simulink model "mngmdl"  (Simulink 7.6)
settings: Solver=FixedStepDiscrete  SolverMode=SingleTasking  StartTime=TIME(1)  StopTime=TIME(end)  FixedStep=SIMSTEP  RelTol=1e-3
model workspace (MAT data in the model file):
  autoc_mdd_data01.esubassyinfo_cfg.cd_brdgname = 'cpsmdlbrg'
  autoc_mdd_data01.esubassyinfo_cfg.cd_exinc = 'on'
  autoc_mdd_data01.esubassyinfo_cfg.cd_chknan = 'on'
  autoc_mdd_data01.esubassyinfo_cfg.cd_geninit = 'on'
  autoc_mdd_data01.esubassyinfo_cfg.cd_fxpimp = 'on'
  autoc_mdd_data01.esubassyinfo_cfg.cd_fixgd = 'on'
  autoc_mdd_data01.esubassyinfo_cfg.cd_models = '.\cpsaflfb.mdl|.\cpsgain.mdl|.\cpsmbtfb.mdl|.\cpsmfb.mdl|.\cpsparam.mdl'
  autoc_mdd_data01.esubassyinfo_cfg.cd_optm_copy = 'off'
  autoc_mdd_data01.esubassyinfo_cfg.cd_optm_nocopy = 'on'
  autoc_mdd_data01.esubassyinfo_cfg.cd_userdefspec = '[-------- 仕様書用 --------]
    | [fram section id]
    | u4g_GSFRAM_CPS_ID
    | [model function]
    | pwon:cpsparam_pwon();
    | pwon:cpsgain_pwon();
    | pwon:cpsmfb_pwon();
    | pwon:cpsaflfb_pwon();
    | pwon:cpsmbtfb_pwon();
    | crank144:cpsparam_crank144();
    | crank144:cpsgain_crank144();
    | crank144:cpsmfb_crank144();
    | crank144:cpsaflfb_crank144();
    | crank144:cpsmbtfb_crank144();
    | [task input]
    | [task output]
    | [output trigger c]
    | [nan recover]
    | [bridge const]
    | [auto counter]
    | [const]
    | [sram]'
  autoc_mdd_data01.esubassyinfo_cfg.cd_userdef_ecuimp : char (value not decoded)
  autoc_mdd_data01.egencode_cfg.cd_stclass_mat = 'rule'
  autoc_mdd_data01.egencode_cfg.cd_option_mode = 'strict'
  autoc_mdd_data01.egencode_cfg.cd_stclass_dsm = 'colored'
  autoc_mdd_data01.egencode_cfg.cd_autoset_simprm = 'on'
  autoc_mdd_data01.egencode_cfg.cd_autoset_mat = 'on'
  autoc_mdd_data01.egencode_cfg.cd_autoset_dsm = 'on'
  autoc_mdd_data01.egencode_cfg.cd_postprocess = 'on'
  autoc_mdd_data01.egencode_cfg.cd_sw_cmatm = 'off'
  autoc_mdd_data01.egencode_cfg.cd_prepro_mdlchk = 'on'
  autoc_mdd_data01.egencode_cfg.cd_cmat_comment = 'on'
  autoc_mdd_data01.egencode_cfg.cd_towscsv_sw = 'off'
  autoc_mdd_data01.egencode_cfg.cd_towscsv_dlg = ''
  autoc_mdd_data01.egencode_cfg.cd_varicodecsv_dlg = ''
  autoc_mdd_data01.egencode_cfg.cd_gencode_lcmat = 'lcmat'
  autoc_mdd_data01.egencode_cfg.cd_option_mode_for_sim = 'off'
  autoc_mdd_data01.egencode_cfg.cd_numexp_opt = 'off'
  autoc_mdd_data01.egencode_cfg.cd_pragmasection = 'cpsmdl_data'
  autoc_mdd_data01.egencode_cfg.cd_returncode_opt = 'off'
  autoc_mdd_data01.egencode_cfg.cd_module_name = 'cpsmdl'
  autoc_mdd_data01.egencode_cfg.cd_expansion_include = '#include "./esrc_cpsmdlbrg.h"'
  autoc_mdd_data01.egencode_cfg.cd_sim_datatype_mode = 'double'
  autoc_mdd_data01.egencode_cfg.cd_mat_cmplsw = 'JEMAT_AUTOC == u1g_EJCC_USE'
  autoc_mdd_data01.egencode_cfg.cd_mon_cmplsw = 'JEMAT_AUTOC == u1g_EJCC_USE'
  autoc_mdd_data01.evaluetows_cfg.cd_ejccpath = ''
  autoc_mdd_data01.evaluetows_cfg.cd_valuews_path = ''
  autoc_mdd_data01.a_cst = []
  autoc_mdd_data01.SIMSTEP = []
  autoc_mdd_data01.MAX_CYL = []
  autoc_mdd_data01.cpsdata_low1 = []
  autoc_mdd_data01.cpsdata_low0 = []
  autoc_mdd_data01.cpsdata_hih1 = []
  autoc_mdd_data01.cpsdata_abs_hih0 = []
  autoc_mdd_data01.cpsdata_hih2 = []
  autoc_mdd_data01.cpsdata_abs_hih1 = []
  autoc_mdd_data01.cpsdata_abs_hih2 = []
  autoc_mdd_data01.cpsdata_hih0 = []
  autoc_mdd_data01.cpsdata_low2 = []
  autoc_mdd_data01.arg_adcn = []
  autoc_mdd_data01.GCIAD_ADCNO0 = []
  autoc_mdd_data01.GACPSCRNK_5CA4CYCLE = []
  autoc_mdd_data01.ON = []
  autoc_mdd_data01.geadd_gepim = []
  autoc_mdd_data01.geadd_gevg = []
  autoc_mdd_data01.geadd_gecps1h = []
  autoc_mdd_data01.geadd_gecps2h = []
  autoc_mdd_data01.geadd_gecps3h = []
  autoc_mdd_data01.geadd_gecps4h = []
  autoc_mdd_data01.geadd_gecps1l = []
  autoc_mdd_data01.geadd_gecps2l = []
  autoc_mdd_data01.geadd_gecps3l = []
  autoc_mdd_data01.geadd_gecps4l = []
  autoc_mdd_data01.revtdc = []
  autoc_mdd_data01.gacpscrnk_cps1 = []
  autoc_mdd_data01.gacpscrnk_cps2 = []
  autoc_mdd_data01.gacpscrnk_cps4 = []
  autoc_mdd_data01.gacpscrnk_cps6 = []
  autoc_mdd_data01.gacpscrnk_cps3 = []
  autoc_mdd_data01.gacpscrnk_cps0 = []
  autoc_mdd_data01.gacpscrnk_cps7 = []
  autoc_mdd_data01.gacpscrnk_cps9 = []
  autoc_mdd_data01.gacpscrnk_cps8 = []
  autoc_mdd_data01.gacpscrnk_cps5 = []
  autoc_mdd_data01.gacpscrnk_cps_idx1 = []
  autoc_mdd_data01.gacpscrnk_cps_idx2 = []
  autoc_mdd_data01.gacpscrnk_cps_result = []
  autoc_mdd_data01.Parameter145 = []
  autoc_mdd_data01.DSM405 = []
  autoc_mdd_data01.DSM406 = []
  autoc_mdd_data01.DSM407 = []
  autoc_mdd_data01.DSM408 = []
  autoc_mdd_data01.DSM409 = []
  autoc_mdd_data01.DSM410 = []
  autoc_mdd_data01.DSM411 = []
  autoc_mdd_data01.DSM412 = []
  autoc_mdd_data01.DSM413 = []
  autoc_mdd_data01.DSM414 = []
  autoc_mdd_data01.DSM39 = []
  autoc_mdd_data01.DSM51 = []
  autoc_mdd_data01.DSM53 = []
  autoc_mdd_data01.DSM62 = []
  autoc_mdd_data01.DSM72 = []
  autoc_mdd_data01.DSM77 = []
  autoc_mdd_data01.DSM79 = []
  autoc_mdd_data01.DSM80 = []
  autoc_mdd_data01.DSM81 = []
values from neighbouring files (symbols this model uses):
  SIMSTEP = 0.0001024    [scr_simdata_all.mat]
Description:
  | AutoCodeGenerator:Version 1.01.A;
settings Model: autoc_cdm_savetype=ModelWorkspace  autoc_cdm_name=autoc_mdd_data01  autoc_current_model=mngmdl  autoc_dsminitmode=spec  Creator=905900  LastModifiedBy=fukudak
settings OptimizationCC: InlineParams=on  InlineInvariantSignals=on  UseTempVars=on  InitFltsAndDblsToZero=on  OptimizeModelRefInitCode=on  LifeSpan=1
settings DebuggingCC: ConsistencyChecking=warning  ArrayBoundsChecking=warning  SignalInfNanChecking=warning  AlgebraicLoopMsg=error  SaveWithParameterizedLinksMsg=none  CheckExecutionContextPreStartOutputMsg=on  CheckExecutionContextRuntimeOutputMsg=on  TimeAdjustmentMsg=warning  SolverPrmCheckMsg=none  InheritedTsInSrcMsg=none  MultiTaskDSMMsg=warning  SingleTaskRateTransMsg=warning  TasksWithSamePriorityMsg=none  IntegerOverflowMsg=error  VectorMatrixConversionMsg=warning  UnconnectedInputMsg=error  UnconnectedOutputMsg=error  UnconnectedLineMsg=error  UniqueDataStoreMsg=error  BusObjectLabelMismatch=error  RootOutportRequireBusObject=error  ModelReferenceIOMsg=warning  ModelReferenceIOMismatchMessage=warning  StrictBusMsg=Warning
settings HardwareCC: ProdIntDivRoundTo=Floor  ProdEndianess=LittleEndian  ProdHWDeviceType=Specified  TargetHWDeviceType=32-bit Generic  ProdEqTarget=off
settings ModelReferenceCC: ModelReferenceNumInstancesAllowed=Single
settings RTWCC: SystemTargetFile=ert.tlc  GenCodeOnly=on  TemplateMakefile=ert_default_tmf  Description=Real-Time Workshop Embedded Coder (no auto configuration)  RTWVerbose=off  ProcessScript=ert_make_rtw_hook
settings CodeAppCC: ForceParamTrailComments=on  IgnoreCustomStorageClasses=off
settings ERTTargetCC: TargetFcnLib=ansi_tfl_tmw.mat  MultiwordLength=2048  GenerateSampleERTMain=on  InlinedParameterPlacement=NonHierarchical  ERTCustomFileTemplate=example_file_process.tlc  ConvertIfToSwitch=off

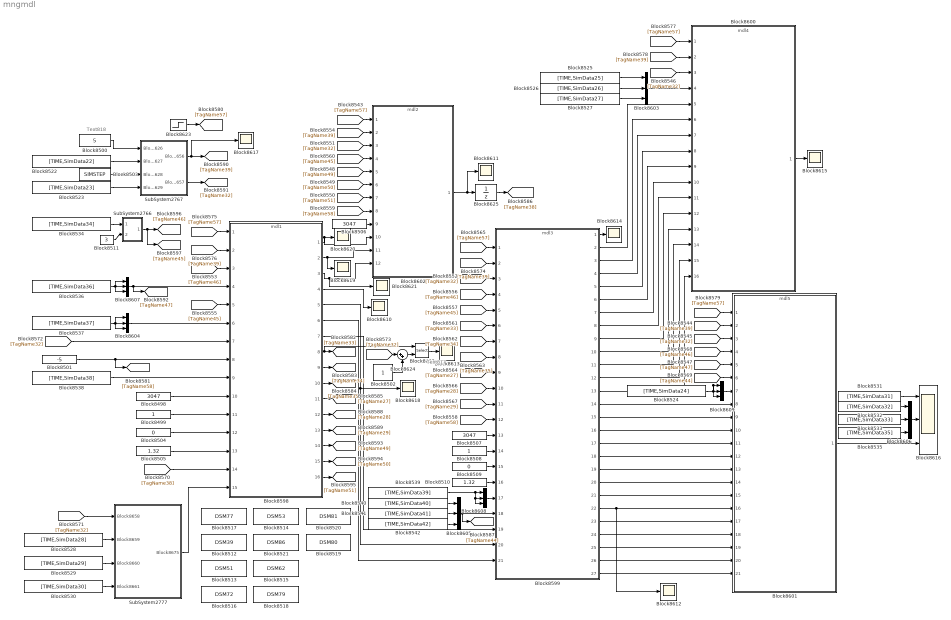
== system mngmdl ==
  note: Text818
  note: Text817
  Block8498 : Constant  Value=3047  OutDataTypeStr=double  SampleTime=SIMSTEP
  Block8499 : Constant  OutDataTypeStr=double  SampleTime=SIMSTEP
  Block8500 : Constant  Value=5  OutDataTypeStr=double  SampleTime=-1
  Block8501 : Constant  Value=-5  OutDataTypeStr=double  SampleTime=SIMSTEP
  Block8502 : Constant  OutDataTypeStr=double  SampleTime=-1
  Block8503 : Constant  Value=SIMSTEP  OutDataTypeStr=double  SampleTime=-1
  Block8504 : Constant  Value=0  OutDataTypeStr=double  SampleTime=SIMSTEP
  Block8505 : Constant  Value=1.32  OutDataTypeStr=double  SampleTime=SIMSTEP
  Block8506 : Constant  Value=3047  OutDataTypeStr=double  SampleTime=-1
  Block8507 : Constant  Value=3047  OutDataTypeStr=double  SampleTime=SIMSTEP
  Block8508 : Constant  OutDataTypeStr=double  SampleTime=SIMSTEP
  Block8509 : Constant  Value=0  OutDataTypeStr=double  SampleTime=SIMSTEP
  Block8510 : Constant  Value=1.32  OutDataTypeStr=double  SampleTime=SIMSTEP
  Block8511 : Constant  Value=3  OutDataTypeStr=double  SampleTime=-1
  Block8512 : DataStoreMemory  DataStoreName=DSM39  InitialValue=[0 0 0 0 0 0 0 0 0 0 0 0 0 0 0 0 0 0 0 0 0 0 0 0 0 0 0 0 0 0 0 0 0 0 0 0 0 0 0 0 0 0 0 0 0 0 0 0 0 0 0 0 0 0 0 0 0 0 0 0 0 0 0 0 0 0 0 0 0 0 0 0 0 0 0 0 0 0 0 0 0 0 0 0 0 0 0 0 0 0 0 0 0 0 0 0 0 0 0 0 0 0 0 0 0 0 0 0 0 0 0 0 0 0 0 0 0 0 0 0 0 0 0 0 0 0 0 0 0 0 0 0 0 0 0 0 0 0 0 0 0 0 0 0]  OutDataTypeStr=double
  Block8513 : DataStoreMemory  DataStoreName=DSM51  InitialValue=[0 0 0 0 0 0 0 0 0 0 0 0 0 0 0 0 0 0 0 0 0 0 0 0 0 0 0 0 0 0 0 0 0 0 0 0 0 0 0 0 0 0 0 0 0 0 0 0 0 0 0 0 0 0 0 0 0 0 0 0 0 0 0 0 0 0 0 0 0 0 0 0 0 0 0 0 0 0 0 0 0 0 0 0 0 0 0 0 0 0 0 0 0 0 0 0 0 0 0 0 0 0 0 0 0 0 0 0 0 0 0 0 0 0 0 0 0 0 0 0 0 0 0 0 0 0 0 0 0 0 0 0 0 0 0 0 0 0 0 0 0 0 0 0]  OutDataTypeStr=double
  Block8514 : DataStoreMemory  DataStoreName=DSM53  InitialValue=[0 0 0 0 0 0 0 0 0 0 0 0 0 0 0 0 0 0 0 0 0 0 0 0 0 0 0 0 0 0 0 0 0 0 0 0 0 0 0 0 0 0 0 0 0 0 0 0 0 0 0 0 0 0 0 0 0 0 0 0 0 0 0 0 0 0 0 0 0 0 0 0 0 0 0 0 0 0 0 0 0 0 0 0 0 0 0 0 0 0 0 0 0 0 0 0 0 0 0 0 0 0 0 0 0 0 0 0 0 0 0 0 0 0 0 0 0 0 0 0 0 0 0 0 0 0 0 0 0 0 0 0 0 0 0 0 0 0 0 0 0 0 0 0]  OutDataTypeStr=double
  Block8515 : DataStoreMemory  DataStoreName=DSM62  InitialValue=[0 0 0 0 0 0 0 0 0 0 0 0 0 0 0 0 0 0 0 0 0 0 0 0 0 0 0 0 0 0 0 0 0 0 0 0 0 0 0 0 0 0 0 0 0 0 0 0 0 0 0 0 0 0 0 0 0 0 0 0 0 0 0 0 0 0 0 0 0 0 0 0 0 0 0 0 0 0 0 0 0 0 0 0 0 0 0 0 0 0 0 0 0 0 0 0 0 0 0 0 0 0 0 0 0 0 0 0 0 0 0 0 0 0 0 0 0 0 0 0 0 0 0 0 0 0 0 0 0 0 0 0 0 0 0 0 0 0 0 0 0 0 0 0]  OutDataTypeStr=double
  Block8516 : DataStoreMemory  DataStoreName=DSM72  InitialValue=[0 0 0 0 0 0 0 0 0 0 0 0 0 0 0 0 0 0 0 0 0 0 0 0 0 0 0 0 0 0 0 0 0 0 0 0 0 0 0 0 0 0 0 0 0 0 0 0 0 0 0 0 0 0 0 0 0 0 0 0 0 0 0 0 0 0 0 0 0 0 0 0 0 0 0 0 0 0 0 0 0 0 0 0 0 0 0 0 0 0 0 0 0 0 0 0 0 0 0 0 0 0 0 0 0 0 0 0 0 0 0 0 0 0 0 0 0 0 0 0 0 0 0 0 0 0 0 0 0 0 0 0 0 0 0 0 0 0 0 0 0 0 0 0]  OutDataTypeStr=double
  Block8517 : DataStoreMemory  DataStoreName=DSM77  InitialValue=[0 0 0 0 0 0 0 0 0 0 0 0 0 0 0 0 0 0 0 0 0 0 0 0 0 0 0 0 0 0 0 0 0 0 0 0 0 0 0 0 0 0 0 0 0 0 0 0 0 0 0 0 0 0 0 0 0 0 0 0 0 0 0 0 0 0 0 0 0 0 0 0 0 0 0 0 0 0 0 0 0 0 0 0 0 0 0 0 0 0 0 0 0 0 0 0 0 0 0 0 0 0 0 0 0 0 0 0 0 0 0 0 0 0 0 0 0 0 0 0 0 0 0 0 0 0 0 0 0 0 0 0 0 0 0 0 0 0 0 0 0 0 0 0]  OutDataTypeStr=double
  Block8518 : DataStoreMemory  DataStoreName=DSM79  InitialValue=[0 0 0 0 0 0 0 0 0 0 0 0 0 0 0 0 0 0 0 0 0 0 0 0 0 0 0 0 0 0 0 0 0 0 0 0 0 0 0 0 0 0 0 0 0 0 0 0 0 0 0 0 0 0 0 0 0 0 0 0 0 0 0 0 0 0 0 0 0 0 0 0 0 0 0 0 0 0 0 0 0 0 0 0 0 0 0 0 0 0 0 0 0 0 0 0 0 0 0 0 0 0 0 0 0 0 0 0 0 0 0 0 0 0 0 0 0 0 0 0 0 0 0 0 0 0 0 0 0 0 0 0 0 0 0 0 0 0 0 0 0 0 0 0]  OutDataTypeStr=double
  Block8519 : DataStoreMemory  DataStoreName=DSM80  InitialValue=[0 0 0 0 0 0 0 0 0 0 0 0 0 0 0 0 0 0 0 0 0 0 0 0 0 0 0 0 0 0 0 0 0 0 0 0 0 0 0 0 0 0 0 0 0 0 0 0 0 0 0 0 0 0 0 0 0 0 0 0 0 0 0 0 0 0 0 0 0 0 0 0 0 0 0 0 0 0 0 0 0 0 0 0 0 0 0 0 0 0 0 0 0 0 0 0 0 0 0 0 0 0 0 0 0 0 0 0 0 0 0 0 0 0 0 0 0 0 0 0 0 0 0 0 0 0 0 0 0 0 0 0 0 0 0 0 0 0 0 0 0 0 0 0]  OutDataTypeStr=double
  Block8520 : DataStoreMemory  DataStoreName=DSM81  InitialValue=[0 0 0 0 0 0 0 0 0 0 0 0 0 0 0 0 0 0 0 0 0 0 0 0 0 0 0 0 0 0 0 0 0 0 0 0 0 0 0 0 0 0 0 0 0 0 0 0 0 0 0 0 0 0 0 0 0 0 0 0 0 0 0 0 0 0 0 0 0 0 0 0 0 0 0 0 0 0 0 0 0 0 0 0 0 0 0 0 0 0 0 0 0 0 0 0 0 0 0 0 0 0 0 0 0 0 0 0 0 0 0 0 0 0 0 0 0 0 0 0 0 0 0 0 0 0 0 0 0 0 0 0 0 0 0 0 0 0 0 0 0 0 0 0]  OutDataTypeStr=double
  Block8521 : DataStoreMemory  DataStoreName=DSM86  InitialValue=[0 0 0 0 0 0 0 0 0 0 0 0 0 0 0 0 0 0 0 0 0 0 0 0 0 0 0 0 0 0 0 0 0 0 0 0 0 0 0 0 0 0 0 0 0 0 0 0 0 0 0 0 0 0 0 0 0 0 0 0 0 0 0 0 0 0 0 0 0 0 0 0 0 0 0 0 0 0 0 0 0 0 0 0 0 0 0 0 0 0 0 0 0 0 0 0 0 0 0 0 0 0 0 0 0 0 0 0 0 0 0 0 0 0 0 0 0 0 0 0 0 0 0 0 0 0 0 0 0 0 0 0 0 0 0 0 0 0 0 0 0 0 0 0]  OutDataTypeStr=double
  Block8522 : FromWorkspace  VariableName=[TIME,SimData22]  SampleTime=SIMSTEP
  Block8523 : FromWorkspace  VariableName=[TIME,SimData23]  SampleTime=SIMSTEP  Interpolate=off  OutputAfterFinalValue=Holding final value
  Block8524 : FromWorkspace  VariableName=[TIME,SimData24]  SampleTime=SIMSTEP
  Block8525 : FromWorkspace  VariableName=[TIME,SimData25]  SampleTime=SIMSTEP
  Block8526 : FromWorkspace  VariableName=[TIME,SimData26]  SampleTime=SIMSTEP
  Block8527 : FromWorkspace  VariableName=[TIME,SimData27]  SampleTime=SIMSTEP
  Block8528 : FromWorkspace  VariableName=[TIME,SimData28]  SampleTime=SIMSTEP
  Block8529 : FromWorkspace  VariableName=[TIME,SimData29]  SampleTime=SIMSTEP
  Block8530 : FromWorkspace  VariableName=[TIME,SimData30]  SampleTime=SIMSTEP
  Block8531 : FromWorkspace  VariableName=[TIME,SimData31]  SampleTime=SIMSTEP
  Block8532 : FromWorkspace  VariableName=[TIME,SimData32]  SampleTime=SIMSTEP
  Block8533 : FromWorkspace  VariableName=[TIME,SimData33]  SampleTime=SIMSTEP
  Block8534 : FromWorkspace  VariableName=[TIME,SimData34]  SampleTime=SIMSTEP
  Block8535 : FromWorkspace  VariableName=[TIME,SimData35]  SampleTime=SIMSTEP
  Block8536 : FromWorkspace  VariableName=[TIME,SimData36]  SampleTime=SIMSTEP
  Block8537 : FromWorkspace  VariableName=[TIME,SimData37]  SampleTime=SIMSTEP
  Block8538 : FromWorkspace  VariableName=[TIME,SimData38]  SampleTime=SIMSTEP
  Block8539 : FromWorkspace  VariableName=[TIME,SimData39]  SampleTime=SIMSTEP
  Block8540 : FromWorkspace  VariableName=[TIME,SimData40]  SampleTime=SIMSTEP
  Block8541 : FromWorkspace  VariableName=[TIME,SimData41]  SampleTime=SIMSTEP
  Block8542 : FromWorkspace  VariableName=[TIME,SimData42]  SampleTime=SIMSTEP
  Block8598 : ModelReference  Priority=2  ModelNameDialog=mdl1  SimulationMode=Normal  ModelReferenceVersion=1.40  CopyOfModelName=mdl1
      settings: AttributesFormatString=Attribute2295
  Block8599 : ModelReference  Priority=4  ModelNameDialog=mdl3  SimulationMode=Normal  ModelReferenceVersion=1.21  CopyOfModelName=mdl3
      settings: AttributesFormatString=Attribute2296
  Block8600 : ModelReference  Priority=5  ModelNameDialog=mdl4  SimulationMode=Normal  ModelReferenceVersion=1.15  CopyOfModelName=mdl4
      settings: AttributesFormatString=Attribute2297
  Block8601 : ModelReference  Priority=6  ModelNameDialog=mdl5  SimulationMode=Normal  ModelReferenceVersion=1.17  CopyOfModelName=mdl5
      settings: AttributesFormatString=Attribute2298
  Block8602 : ModelReference  Priority=3  ModelNameDialog=mdl2  SimulationMode=Normal  ModelReferenceVersion=1.14  CopyOfModelName=mdl2
      settings: AttributesFormatString=Attribute2299
  Block{8603..8609} (7 alike) : Mux  Inputs=3
  Block{8610..8615,8617..8621} (11 alike) : Scope
      Block8611 settings: YMin=0.95  YMax=1.05
      Block8612 settings: YMin=-0.00475  YMax=-0.0015  SaveName=ScopeData2
      Block8613 settings: YMin=0.125  YMax=0.65  SaveName=ScopeData9
      Block8614 settings: YMin=-1  YMax=1  SaveName=ScopeData10
      Block8615 settings: SaveName=ScopeData11
      Block8617 settings: YMin=0  YMax=1  SaveName=ScopeData4
      Block8618 settings: SaveName=ScopeData5
      Block8619 settings: TimeRange=42.74809160305345  YMin=-0.4345238095238095  YMax=0.2202380952380953  SaveName=ScopeData6
      Block8620 settings: SaveName=ScopeData7
      Block8621 settings: SaveName=ScopeData8
  Block8616 : Scope  NumInputPorts=3
      settings: TimeRange=70  YMin=400~0.8~4.5  YMax=2200~1.8~5.5  SaveName=ScopeData3
  Block8622 : Selector  IndexOptions=Index vector (port)  Indices=[1 3]  OutputSizes=1
  Block8623 : Step  Time=SIMSTEP  SampleTime=SIMSTEP
  Block8624 : Sum  Inputs=|++  OutDataTypeStr=double  RndMeth=Zero  SaturateOnIntegerOverflow=on  InputSameDT=on
  Block8625 : UnitDelay  SampleTime=-1
  SubSystem2766 : Subsystem
  SubSystem2767 : Subsystem
  SubSystem2777 : Subsystem  RTWFileName=eset_real
      settings: AttributesFormatString=Attribute2311  RTWFcnNameOpts=Use subsystem name
  wires:
  Block8598/4 -> Block8610/1
  Block8599/1 -> Block8614/1
  Block8600/1 -> Block8615/1
  Block8599/2 -> Block8600/5
  Block8599/3 -> Block8600/6
  Block8599/4 -> Block8600/7
  Block8599/5 -> Block8600/8
  Block8599/6 -> Block8600/9
  Block8599/7 -> Block8600/10
  Block8599/8 -> Block8600/11
  Block8599/9 -> Block8600/12
  Block8599/10 -> Block8600/13
  Block8599/11 -> Block8600/14
  Block8599/12 -> Block8600/15
  Block8599/13 -> Block8600/16
  Block8599/14 -> Block8601/8
  Block8599/15 -> Block8601/9
  Block8599/16 -> Block8601/10
  Block8599/17 -> Block8601/11
  Block8599/18 -> Block8601/12
  Block8599/19 -> Block8601/13
  Block8599/20 -> Block8601/14
  Block8599/21 -> Block8601/15
  Block8599/22 -> Block8601/16, Block8612/1
  Block8599/23 -> Block8601/17
  Block8599/24 -> Block8601/18
  Block8599/25 -> Block8601/19
  Block8599/26 -> Block8601/20
  Block8599/27 -> Block8601/21
  Block8598/1 -> Block8620/1, Block8602/10
  Block8598/2 -> Block8619/1, Block8602/11
  Block8598/3 -> Block8602/12, Block8621/1
  Block8598/7 -> Block8599/19
  Block8598/5 -> Block8599/20, Block8618/1
  Block8598/6 -> Block8599/21
  Block8607/1 -> Block8598/4, [TagName47]
  Block8604/1 -> Block8598/6
  Block8501/1 -> [TagName58], Block8598/8
  Block8506/1 -> Block8602/9
  [TagName58] -> Block8602/8
  Block8623/1 -> [TagName57]
  [TagName57] -> Block8598/1
  [TagName39] -> Block8598/2
  [TagName57] -> Block8602/1
  [TagName39] -> Block8602/2
  [TagName57] -> Block8599/1
  [TagName39] -> Block8599/2
  [TagName57] -> Block8600/1
  [TagName39] -> Block8600/2
  Block8525/1 -> Block8603/1
  Block8526/1 -> Block8603/2
  Block8527/1 -> Block8603/3
  Block8603/1 -> Block8600/4
  [TagName57] -> Block8601/1
  [TagName39] -> Block8601/2
  [TagName32] -> Block8601/3
  [TagName32] -> Block8600/3
  [TagName44] -> Block8601/6
  [TagName47] -> Block8601/5
  [TagName49] -> Block8602/5
  [TagName51] -> Block8602/7
  [TagName50] -> Block8602/6
  [TagName32] -> Block8602/3
  [TagName32] -> Block8599/3
  Block8534/1 -> SubSystem2766/1(Scalar)
  [TagName46] -> Block8598/3
  [TagName45] -> Block8598/5
  [TagName46] -> Block8599/4
  [TagName45] -> Block8599/5
  [TagName58] -> Block8599/12
  Block8507/1 -> Block8599/13
  Block8508/1 -> Block8599/14
  Block8509/1 -> Block8599/15
  Block8510/1 -> Block8599/16
  [TagName45] -> Block8602/4
  Block8540/1 -> Block8605/1
  Block8541/1 -> Block8605/2
  Block8542/1 -> Block8605/3
  Block8605/1 -> Block8599/18, [TagName44]
  [TagName33] -> Block8599/6
  [TagName35] -> Block8599/8
  [TagName34] -> Block8599/7
  [TagName27] -> Block8599/9
  [TagName28] -> Block8599/10
  [TagName29] -> Block8599/11
  [TagName46] -> Block8601/4
  SubSystem2766/1(Vector) -> [TagName46], [TagName45]
  Block8511/1 -> SubSystem2766/2(Width)
  Block8537/1 -> Block8604/3, Block8604/1, Block8604/2
  Block8536/1 -> Block8607/2, Block8607/3, Block8607/1
  Block8608/1 -> Block8599/17
  Block8539/1 -> Block8608/1, Block8608/2, Block8608/3
  Block8609/1 -> Block8601/7
  Block8524/1 -> Block8609/3, Block8609/2, Block8609/1
  Block8602/1 -> Block8625/1, Block8611/1
  Block8625/1 -> [TagName38]
  [TagName32] -> SubSystem2777/1(Block8658)
  Block8528/1 -> SubSystem2777/2(Block8659)
  Block8529/1 -> SubSystem2777/3(Block8660)
  Block8530/1 -> SubSystem2777/4(Block8661)
  [TagName32] -> Block8598/7
  Block8538/1 -> Block8598/9
  Block8498/1 -> Block8598/10
  Block8499/1 -> Block8598/11
  Block8504/1 -> Block8598/12
  Block8505/1 -> Block8598/13
  [TagName38] -> Block8598/14
  SubSystem2777/1(Block8675) -> Block8598/15
  Block8598/8 -> [TagName33], Block8622/1
  Block8598/9 -> [TagName34]
  Block8598/16 -> [TagName51]
  Block8598/15 -> [TagName50]
  Block8598/14 -> [TagName49]
  Block8598/13 -> [TagName29]
  Block8598/12 -> [TagName28]
  Block8598/11 -> [TagName27]
  Block8598/10 -> [TagName35]
  Block8622/1 -> Block8613/1
  [TagName32] -> Block8624/1
  Block8624/1 -> Block8622/2
  Block8502/1 -> Block8624/2
  Block8522/1 -> SubSystem2767/2(Block8627)
  Block8503/1 -> SubSystem2767/3(Block8628)
  SubSystem2767/2(Block8657) -> [TagName32]
  Block8523/1 -> SubSystem2767/4(Block8629)
  Block8500/1 -> SubSystem2767/1(Block8626)
  SubSystem2767/1(Block8656) -> [TagName39], Block8617/1
  Block8532/1 -> Block8606/1
  Block8533/1 -> Block8606/2
  Block8535/1 -> Block8606/3
  Block8531/1 -> Block8616/1
  Block8606/1 -> Block8616/2
  Block8601/1 -> Block8616/3

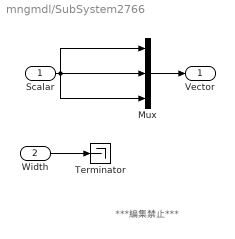
== system mngmdl/SubSystem2766 ==
  note: ***編集禁止***
  Scalar : Inport
  Width : Inport  Port=2
  Mux : Mux  Inputs=3
  Terminator : Terminator
  Vector : Outport
  wires:
  Width/1 -> Terminator/1
  Mux/1 -> Vector/1
  Scalar/1 -> Mux/1, Mux/2, Mux/3

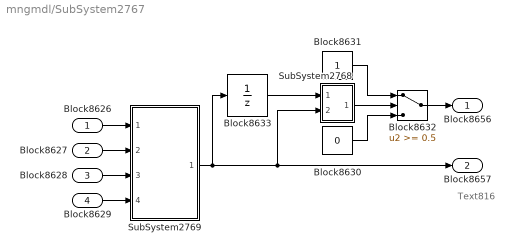
== system mngmdl/SubSystem2767 ==
  note: Text816
  Block8626 : Inport
  Block8627 : Inport  Port=2
  Block8628 : Inport  Port=3
  Block8629 : Inport  Port=4
  Block8630 : Constant  Value=0  OutDataTypeStr=double  SampleTime=-1
  Block8631 : Constant  OutDataTypeStr=double  SampleTime=-1
  Block8632 : Switch  Threshold=0.5  RndMeth=Zero  SaturateOnIntegerOverflow=on  InputSameDT=on
  Block8633 : UnitDelay  SampleTime=-1
  SubSystem2768 : Subsystem
  SubSystem2769 : Subsystem
  Block8656 : Outport
  Block8657 : Outport  Port=2
  wires:
  SubSystem2769/1(Block8655) -> Block8633/1, Block8657/1, SubSystem2768/2(In2)
  Block8633/1 -> SubSystem2768/1(In1)
  SubSystem2768/1(Out1) -> Block8632/2
  Block8631/1 -> Block8632/1
  Block8630/1 -> Block8632/3
  Block8632/1 -> Block8656/1
  Block8627/1 -> SubSystem2769/2(Block8635)
  Block8628/1 -> SubSystem2769/3(Block8636)
  Block8629/1 -> SubSystem2769/4(Block8637)
  Block8626/1 -> SubSystem2769/1(Block8634)

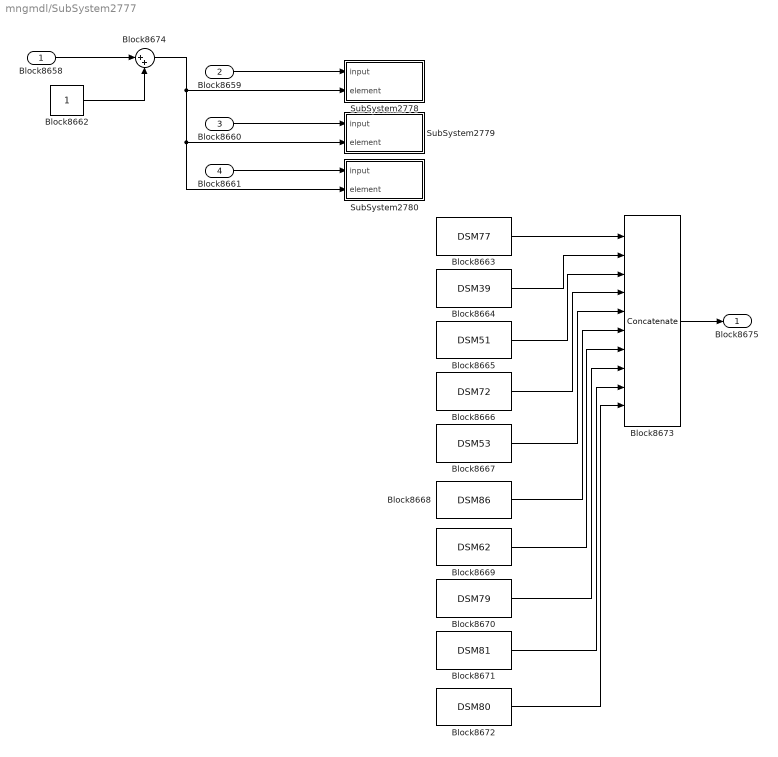
== system mngmdl/SubSystem2777 ==
  Block8658 : Inport
  Block8659 : Inport  Port=2
  Block8660 : Inport  Port=3
  Block8661 : Inport  Port=4
  Block8662 : Constant  OutDataTypeStr=double  SampleTime=-1
  Block8663 : DataStoreRead  DataStoreName=DSM77
  Block8664 : DataStoreRead  DataStoreName=DSM39
  Block8665 : DataStoreRead  DataStoreName=DSM51
  Block8666 : DataStoreRead  DataStoreName=DSM72
  Block8667 : DataStoreRead  DataStoreName=DSM53
  Block8668 : DataStoreRead  DataStoreName=DSM86
  Block8669 : DataStoreRead  DataStoreName=DSM62
  Block8670 : DataStoreRead  DataStoreName=DSM79
  Block8671 : DataStoreRead  DataStoreName=DSM81
  Block8672 : DataStoreRead  DataStoreName=DSM80
  Block8673 : Concatenate  NumInputs=10  Mode=Multidimensional array  ConcatenateDimension=2
  Block8674 : Sum  Inputs=|++  OutDataTypeStr=double  RndMeth=Zero  SaturateOnIntegerOverflow=on  InputSameDT=on
  SubSystem2778 : Subsystem  TreatAsAtomicUnit=on  mask(***ATC.DSWVEC***){bd_version=1.01.A, r0=DSM77, r1=-1, r2=, r3=, r4=, r5=, r6=, r7=, r8=, r9=, c0=, c1=, c2=, c3=, c4=, c5=, c6=, c7=, c8=, c9=}
      mask prompts: bd_version "Version"
      mask help: これはAutoCからのブロックです．編集禁止．
      settings: OpenFcn=warndlg('変更禁止!');
      mask Help: web(ui_blockhelpmng(gcb));
      mask Display: disp('ATC.DSRVEC')
  SubSystem2779 : Subsystem  TreatAsAtomicUnit=on  mask(***ATC.DSWVEC***){bd_version=1.01.A, r0=DSM39, r1=-1, r2=, r3=, r4=, r5=, r6=, r7=, r8=, r9=, c0=, c1=, c2=, c3=, c4=, c5=, c6=, c7=, c8=, c9=}
      mask prompts: bd_version "Version"
      mask help: これはAutoCからのブロックです．編集禁止．
      settings: OpenFcn=warndlg('変更禁止!');
      mask Help: web(ui_blockhelpmng(gcb));
      mask Display: disp('ATC.DSRVEC')
  SubSystem2780 : Subsystem  TreatAsAtomicUnit=on  mask(***ATC.DSWVEC***){bd_version=1.01.A, r0=DSM51, r1=-1, r2=, r3=, r4=, r5=, r6=, r7=, r8=, r9=, c0=, c1=, c2=, c3=, c4=, c5=, c6=, c7=, c8=, c9=}
      mask prompts: bd_version "Version"
      mask help: これはAutoCからのブロックです．編集禁止．
      settings: OpenFcn=warndlg('変更禁止!');
      mask Help: web(ui_blockhelpmng(gcb));
      mask Display: disp('ATC.DSRVEC')
  Block8675 : Outport
  wires:
  Block8662/1 -> Block8674/2
  Block8658/1 -> Block8674/1
  Block8659/1 -> SubSystem2778/1(input)
  Block8660/1 -> SubSystem2779/1(input)
  Block8661/1 -> SubSystem2780/1(input)
  Block8674/1 -> SubSystem2780/2(element), SubSystem2779/2(element), SubSystem2778/2(element)
  Block8663/1 -> Block8673/1
  Block8664/1 -> Block8673/2
  Block8665/1 -> Block8673/3
  Block8673/1 -> Block8675/1
  Block8666/1 -> Block8673/4
  Block8667/1 -> Block8673/5
  Block8668/1 -> Block8673/6
  Block8669/1 -> Block8673/7
  Block8670/1 -> Block8673/8
  Block8671/1 -> Block8673/9
  Block8672/1 -> Block8673/10

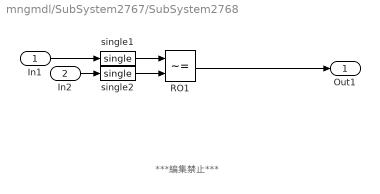
== system mngmdl/SubSystem2767/SubSystem2768 ==
  note: ***編集禁止***
  In1 : Inport
  In2 : Inport  Port=2
  RO1 : RelationalOperator  Operator=~=  InputSameDT=on
  single1 : DataTypeConversion  OutDataTypeStr=single  SaturateOnIntegerOverflow=on  RndMeth=Zero
  single2 : DataTypeConversion  OutDataTypeStr=single  SaturateOnIntegerOverflow=on  RndMeth=Zero
  Out1 : Outport
  wires:
  RO1/1 -> Out1/1
  In2/1 -> single2/1
  In1/1 -> single1/1
  single1/1 -> RO1/1
  single2/1 -> RO1/2

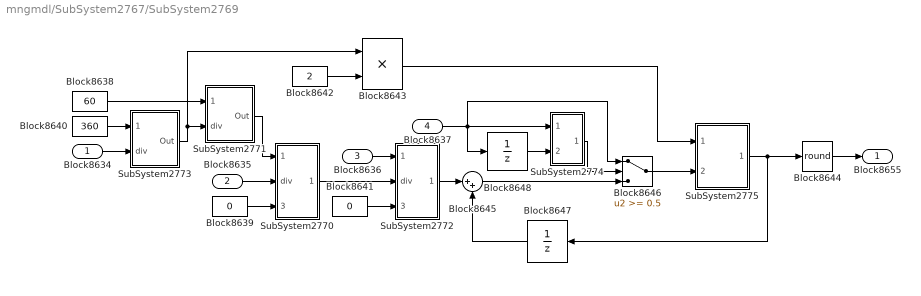
== system mngmdl/SubSystem2767/SubSystem2769 ==
  Block8634 : Inport
  Block8635 : Inport  Port=2
  Block8636 : Inport  Port=3
  Block8637 : Inport  Port=4
  Block8638 : Constant  Value=60  OutDataTypeStr=double  SampleTime=-1
  Block8639 : Constant  Value=0  OutDataTypeStr=double  SampleTime=-1
  Block8640 : Constant  Value=360  OutDataTypeStr=double  SampleTime=-1
  Block8641 : Constant  Value=0  OutDataTypeStr=double  SampleTime=-1
  Block8642 : Constant  Value=2  OutDataTypeStr=double  SampleTime=-1
  Block8643 : Product  Inputs=**  SaturateOnIntegerOverflow=on  RndMeth=Zero  InputSameDT=on  OutDataTypeStr=Inherit: Same as first input
  Block8644 : Rounding  Operator=round
  Block8645 : Sum  Inputs=|++  OutDataTypeStr=double  RndMeth=Zero  SaturateOnIntegerOverflow=on  InputSameDT=on
  Block8646 : Switch  Threshold=0.5  RndMeth=Zero  SaturateOnIntegerOverflow=on  InputSameDT=on
  Block8647 : UnitDelay  SampleTime=-1
  Block8648 : UnitDelay  SampleTime=-1
  SubSystem2770 : Subsystem  TreatAsAtomicUnit=on  mask(***ATC.DIVISION***){bd_version=1.01.A, r0=チェック有り, r1=, r2=, r3=, r4=, r5=, r6=, r7=, r8=, r9=, c0=, c1=, c2=, c3=, c4=, c5=, c6=, c7=, c8=, c9=}
      mask prompts: bd_version "Version"
      mask help: これはAutoCからのブロックです．編集禁止．
      settings: OpenFcn=warndlg('変更禁止!');
      mask Help: web(ui_blockhelpmng(gcb));
  SubSystem2771 : Subsystem  TreatAsAtomicUnit=on  mask(***ATC.DIVISION***){bd_version=1.01.A, r0=チェック無し, r1=, r2=, r3=, r4=, r5=, r6=, r7=, r8=, r9=, c0=, c1=, c2=, c3=, c4=, c5=, c6=, c7=, c8=, c9=}
      mask prompts: bd_version "Version"
      mask help: これはAutoCからのブロックです．編集禁止．
      settings: OpenFcn=warndlg('変更禁止!');
      mask Help: web(ui_blockhelpmng(gcb));
  SubSystem2772 : Subsystem  TreatAsAtomicUnit=on  mask(***ATC.DIVISION***){bd_version=1.01.A, r0=チェック有り, r1=, r2=, r3=, r4=, r5=, r6=, r7=, r8=, r9=, c0=, c1=, c2=, c3=, c4=, c5=, c6=, c7=, c8=, c9=}
      mask prompts: bd_version "Version"
      mask help: これはAutoCからのブロックです．編集禁止．
      settings: OpenFcn=warndlg('変更禁止!');
      mask Help: web(ui_blockhelpmng(gcb));
  SubSystem2773 : Subsystem  TreatAsAtomicUnit=on  mask(***ATC.DIVISION***){bd_version=1.01.A, r0=チェック無し, r1=, r2=, r3=, r4=, r5=, r6=, r7=, r8=, r9=, c0=, c1=, c2=, c3=, c4=, c5=, c6=, c7=, c8=, c9=}
      mask prompts: bd_version "Version"
      mask help: これはAutoCからのブロックです．編集禁止．
      settings: OpenFcn=warndlg('変更禁止!');
      mask Help: web(ui_blockhelpmng(gcb));
  SubSystem2774 : Subsystem
  SubSystem2775 : Subsystem
      settings: RTWSystemCode=Inline
  Block8655 : Outport
  wires:
  Block8647/1 -> Block8645/2
  Block8645/1 -> Block8646/3
  Block8635/1 -> SubSystem2770/2(div)
  Block8639/1 -> SubSystem2770/3(init)
  Block8638/1 -> SubSystem2771/1(mult)
  SubSystem2771/1(Out) -> SubSystem2770/1(mult)
  SubSystem2772/1(Out) -> Block8645/1
  Block8636/1 -> SubSystem2772/1(mult)
  SubSystem2770/1(Out) -> SubSystem2772/2(div)
  Block8641/1 -> SubSystem2772/3(init)
  Block8644/1 -> Block8655/1
  SubSystem2774/1(Out1) -> Block8646/2
  Block8637/1 -> SubSystem2774/1(In1), Block8648/1, Block8646/1
  Block8648/1 -> SubSystem2774/2(In2)
  Block8646/1 -> SubSystem2775/2(Block8650)
  SubSystem2775/1(Block8654) -> Block8644/1, Block8647/1
  Block8640/1 -> SubSystem2773/1(mult)
  Block8634/1 -> SubSystem2773/2(div)
  Block8642/1 -> Block8643/2
  SubSystem2773/1(Out) -> SubSystem2771/2(div), Block8643/1
  Block8643/1 -> SubSystem2775/1(Block8649)

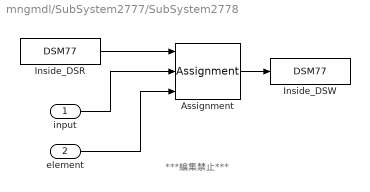
== system mngmdl/SubSystem2777/SubSystem2778 ==
  note: ***編集禁止***
  input : Inport
  element : Inport  Port=2
  Assignment : Assignment  IndexOptions=Index vector (port)  Indices=1  OutputSizes=[1 1]
  Inside_DSR : DataStoreRead  DataStoreName=DSM77
  Inside_DSW : DataStoreWrite  DataStoreName=DSM77
  wires:
  Assignment/1 -> Inside_DSW/1
  Inside_DSR/1 -> Assignment/1
  input/1 -> Assignment/2
  element/1 -> Assignment/3

== system mngmdl/SubSystem2777/SubSystem2779 ==
  note: ***編集禁止***
  input : Inport
  element : Inport  Port=2
  Assignment : Assignment  IndexOptions=Index vector (port)  Indices=1  OutputSizes=[1 1]
  Inside_DSR : DataStoreRead  DataStoreName=DSM39
  Inside_DSW : DataStoreWrite  DataStoreName=DSM39
  wires:
  element/1 -> Assignment/3
  input/1 -> Assignment/2
  Inside_DSR/1 -> Assignment/1
  Assignment/1 -> Inside_DSW/1

== system mngmdl/SubSystem2777/SubSystem2780 ==
  note: ***編集禁止***
  input : Inport
  element : Inport  Port=2
  Assignment : Assignment  IndexOptions=Index vector (port)  Indices=1  OutputSizes=[1 1]
  Inside_DSR : DataStoreRead  DataStoreName=DSM51
  Inside_DSW : DataStoreWrite  DataStoreName=DSM51
  wires:
  Assignment/1 -> Inside_DSW/1
  Inside_DSR/1 -> Assignment/1
  input/1 -> Assignment/2
  element/1 -> Assignment/3

== system mngmdl/SubSystem2767/SubSystem2769/SubSystem2770 ==
  note: ***編集禁止***
  mult : Inport
  div : Inport  Port=2
  init : Inport  Port=3
  Product : Subsystem  TreatAsAtomicUnit=on
      settings: RTWSystemCode=Inline
  Out : Outport
  wires:
  Product/1(Out) -> Out/1
  mult/1 -> Product/1(mult)
  div/1 -> Product/2(div)
  init/1 -> Product/3(init)

== system mngmdl/SubSystem2767/SubSystem2769/SubSystem2771 ==
  note: ***編集禁止***
  mult : Inport
  div : Inport  Port=2
  Product : Product  Inputs=*/  SaturateOnIntegerOverflow=on  RndMeth=Zero  InputSameDT=on  OutDataTypeStr=Inherit: Same as first input
  Out : Outport
  wires:
  Product/1 -> Out/1
  mult/1 -> Product/1
  div/1 -> Product/2

== system mngmdl/SubSystem2767/SubSystem2769/SubSystem2772 ==
  note: ***編集禁止***
  mult : Inport
  div : Inport  Port=2
  init : Inport  Port=3
  Product : Subsystem  TreatAsAtomicUnit=on
      settings: RTWSystemCode=Inline
  Out : Outport
  wires:
  init/1 -> Product/3(init)
  div/1 -> Product/2(div)
  mult/1 -> Product/1(mult)
  Product/1(Out) -> Out/1

== system mngmdl/SubSystem2767/SubSystem2769/SubSystem2773 ==
  note: ***編集禁止***
  mult : Inport
  div : Inport  Port=2
  Product : Product  Inputs=*/  SaturateOnIntegerOverflow=on  RndMeth=Zero  InputSameDT=on  OutDataTypeStr=Inherit: Same as first input
  Out : Outport
  wires:
  div/1 -> Product/2
  mult/1 -> Product/1
  Product/1 -> Out/1

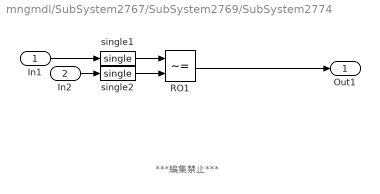
== system mngmdl/SubSystem2767/SubSystem2769/SubSystem2774 ==
  note: ***編集禁止***
  In1 : Inport
  In2 : Inport  Port=2
  RO1 : RelationalOperator  Operator=~=  InputSameDT=on
  single1 : DataTypeConversion  OutDataTypeStr=single  SaturateOnIntegerOverflow=on  RndMeth=Zero
  single2 : DataTypeConversion  OutDataTypeStr=single  SaturateOnIntegerOverflow=on  RndMeth=Zero
  Out1 : Outport
  wires:
  single2/1 -> RO1/2
  single1/1 -> RO1/1
  In1/1 -> single1/1
  In2/1 -> single2/1
  RO1/1 -> Out1/1

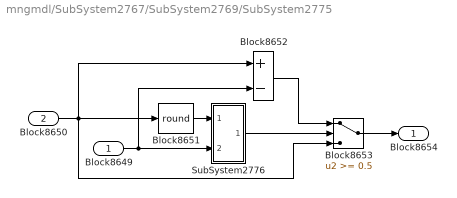
== system mngmdl/SubSystem2767/SubSystem2769/SubSystem2775 ==
  Block8649 : Inport
  Block8650 : Inport  Port=2
  Block8651 : Rounding  Operator=round
  Block8652 : Sum  Inputs=+-  OutDataTypeStr=double  RndMeth=Zero  SaturateOnIntegerOverflow=on  InputSameDT=on
  Block8653 : Switch  Threshold=0.5  RndMeth=Zero  SaturateOnIntegerOverflow=on  InputSameDT=on
  SubSystem2776 : Subsystem
  Block8654 : Outport
  wires:
  Block8650/1 -> Block8652/1, Block8653/3, Block8651/1
  Block8649/1 -> Block8652/2, SubSystem2776/2(In2)
  SubSystem2776/1(Out1) -> Block8653/2
  Block8653/1 -> Block8654/1
  Block8652/1 -> Block8653/1
  Block8651/1 -> SubSystem2776/1(In1)

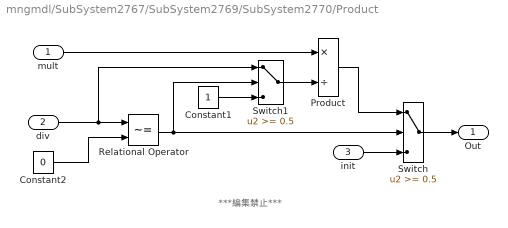
== system mngmdl/SubSystem2767/SubSystem2769/SubSystem2770/Product ==
  note: ***編集禁止***
  mult : Inport
  div : Inport  Port=2
  init : Inport  Port=3
  Constant1 : Constant  OutDataTypeStr=Inherit: Inherit via back propagation
  Constant2 : Constant  Value=0  OutDataTypeStr=Inherit: Inherit via back propagation
  Product : Product  Inputs=*/  SaturateOnIntegerOverflow=on  RndMeth=Zero  InputSameDT=on  OutDataTypeStr=Inherit: Same as first input
  Relational Operator : RelationalOperator  Operator=~=  InputSameDT=on
  Switch : Switch  Threshold=0.5  SaturateOnIntegerOverflow=on  InputSameDT=on
  Switch1 : Switch  Threshold=0.5  SaturateOnIntegerOverflow=on  InputSameDT=on
  Out : Outport
  wires:
  Constant1/1 -> Switch1/3
  Constant2/1 -> Relational Operator/2
  Switch1/1 -> Product/2
  div/1 -> Relational Operator/1, Switch1/1
  Switch/1 -> Out/1
  init/1 -> Switch/3
  Relational Operator/1 -> Switch1/2, Switch/2
  Product/1 -> Switch/1
  mult/1 -> Product/1

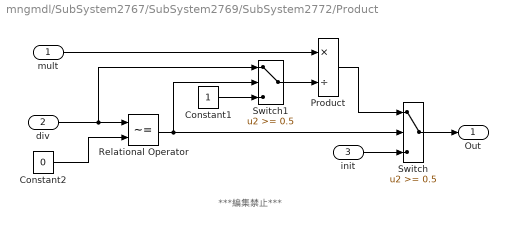
== system mngmdl/SubSystem2767/SubSystem2769/SubSystem2772/Product ==
  note: ***編集禁止***
  mult : Inport
  div : Inport  Port=2
  init : Inport  Port=3
  Constant1 : Constant  OutDataTypeStr=Inherit: Inherit via back propagation
  Constant2 : Constant  Value=0  OutDataTypeStr=Inherit: Inherit via back propagation
  Product : Product  Inputs=*/  SaturateOnIntegerOverflow=on  RndMeth=Zero  InputSameDT=on  OutDataTypeStr=Inherit: Same as first input
  Relational Operator : RelationalOperator  Operator=~=  InputSameDT=on
  Switch : Switch  Threshold=0.5  SaturateOnIntegerOverflow=on  InputSameDT=on
  Switch1 : Switch  Threshold=0.5  SaturateOnIntegerOverflow=on  InputSameDT=on
  Out : Outport
  wires:
  Constant1/1 -> Switch1/3
  Constant2/1 -> Relational Operator/2
  Switch1/1 -> Product/2
  div/1 -> Relational Operator/1, Switch1/1
  Switch/1 -> Out/1
  init/1 -> Switch/3
  Relational Operator/1 -> Switch1/2, Switch/2
  Product/1 -> Switch/1
  mult/1 -> Product/1

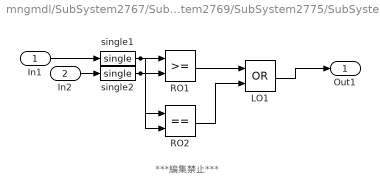
== system mngmdl/SubSystem2767/SubSystem2769/SubSystem2775/SubSystem2776 ==
  note: ***編集禁止***
  In1 : Inport
  In2 : Inport  Port=2
  LO1 : Logic  Operator=OR
  RO1 : RelationalOperator  InputSameDT=on
  RO2 : RelationalOperator  Operator===  InputSameDT=on
  single1 : DataTypeConversion  OutDataTypeStr=single  SaturateOnIntegerOverflow=on  RndMeth=Zero
  single2 : DataTypeConversion  OutDataTypeStr=single  SaturateOnIntegerOverflow=on  RndMeth=Zero
  Out1 : Outport
  wires:
  In2/1 -> single2/1
  In1/1 -> single1/1
  single1/1 -> RO1/1, RO2/1
  single2/1 -> RO1/2, RO2/2
  RO1/1 -> LO1/1
  RO2/1 -> LO1/2
  LO1/1 -> Out1/1
